simulink model "pt8612pllsimple"  (Simulink 5.0)
settings: Solver=ode45  StartTime=0.0  StopTime=10  RelTol=1e-7  AbsTol=1e-10
values from neighbouring files (symbols this model uses):
  C = 680e-9    (= 6.8e-07)    [PT8612PLLinit.m]    (also in PT8612PLLinit_2.m; PT8612PLLinit_3.m; PT8612PLLinit_4.m; colorimetry_rom.m = [[CrCgCb(1) 0 0];[0 CrCgCb(2) 0];[0 0 CrCgCb(3)]])
  fvcxo = 148.5e6/1.001    (= 148351648.352)    [PT8612PLLinit.m]    (also in PT8612PLLinit_2.m; PT8612PLLinit_3.m; PT8612PLLinit_4.m)
  Gi = 1/32    (= 0.03125)    [PT8612PLLinit.m]    (also in PT8612PLLinit_2.m = 0.05)
  Gp = 1/4    (= 0.25)    [PT8612PLLinit.m]    (also in PT8612PLLinit_2.m = 0.025; PT8612PLLinit_4.m = 256)
  Kvcxo = 90e-6    (= 9e-05)    [PT8612PLLinit.m]    (also in PT8612PLLinit_2.m; PT8612PLLinit_3.m; PT8612PLLinit_4.m)
  R = 100e3    (= 100000)    [PT8612PLLinit.m]    (also in PT8612PLLinit_2.m = 220000; PT8612PLLinit_3.m = 82000; PT8612PLLinit_4.m = 200000; combi_signal.m = [R;ones(red_heigth,spl)])
libraries: simulink x1
settings Model: LastModifiedBy=thh

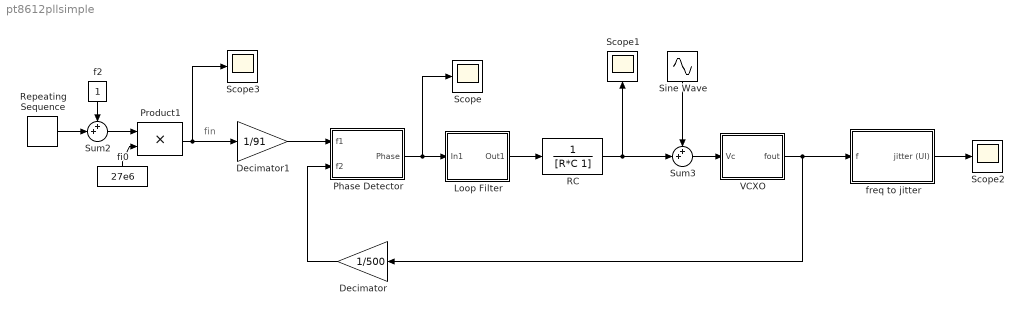
== system pt8612pllsimple ==
  note: fin
  Decimator : Gain  Orientation=left  Gain=1/500  SaturateOnIntegerOverflow=on
  Decimator1 : Gain  Gain=1/91  SaturateOnIntegerOverflow=on
  Loop Filter : Subsystem
  Phase Detector : Subsystem
  Product1 : Product  SaturateOnIntegerOverflow=on
  RC : TransferFcn  Denominator=[R*C 1]
  Repeating Sequence : simulink/Sources/Repeating Sequence  rep_seq_t=[0 1 1 10]  rep_seq_y=[0 0 1 1]*0
  Scope{,1..3} (4 alike) : Scope
      Scope settings: YMin=5.55112e-017  YMax=1.9
      Scope1 settings: Orientation=up  TimeRange=10  YMin=-0.35  YMax=0.2
      Scope2 settings: TimeRange=10  YMin=-1  YMax=0.8  SaveName=ScopeData3
      Scope3 settings: YMin=5.55112e-017  YMax=1.9  SaveName=ScopeData4
  Sine Wave : Sin  Orientation=down  Frequency=80  SampleTime=0
  Sum2 : Sum  Inputs=++|  SaturateOnIntegerOverflow=on
  Sum3 : Sum  Inputs=++|  SaturateOnIntegerOverflow=on
  VCXO : Subsystem
  f2 : Constant  Orientation=down
  fi0 : Constant  Orientation=up  Value=27e6
  freq to jitter : Subsystem
  wires:
  Phase Detector/1(Phase) -> Scope/1, Loop Filter/1(In1)
  VCXO/1(fout) -> Decimator/1, freq to jitter/1(f)
  Product1/1 -> Decimator1/1, Scope3/1
  fi0/1 -> Product1/2
  f2/1 -> Sum2/1
  Sum2/1 -> Product1/1
  Repeating Sequence/1 -> Sum2/2
  Decimator/1 -> Phase Detector/2(f2)
  Decimator1/1 -> Phase Detector/1(f1)
  Loop Filter/1(Out1) -> RC/1
  RC/1 -> Scope1/1, Sum3/2
  freq to jitter/1(jitter (UI)) -> Scope2/1
  Sum3/1 -> VCXO/1(Vc)
  Sine Wave/1 -> Sum3/1

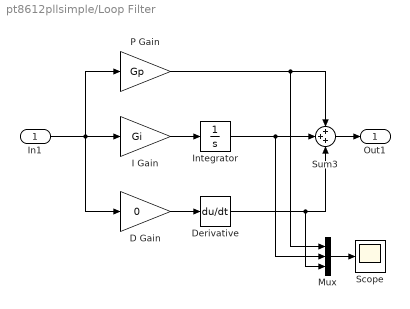
== system pt8612pllsimple/Loop Filter ==
  In1 : Inport
  D Gain : Gain  Gain=0  SaturateOnIntegerOverflow=on
  Derivative : Derivative
  I Gain : Gain  Gain=Gi  SaturateOnIntegerOverflow=on
  Integrator : Integrator
  Mux : Mux  Inputs=3
  P Gain : Gain  Gain=Gp  SaturateOnIntegerOverflow=on
  Scope : Scope
      settings: YMin=0  YMax=0.85  SaveName=ScopeData2
  Sum3 : Sum  Inputs=+++  SaturateOnIntegerOverflow=on
  Out1 : Outport
  wires:
  I Gain/1 -> Integrator/1
  P Gain/1 -> Sum3/1, Mux/1
  In1/1 -> I Gain/1, P Gain/1, D Gain/1
  Sum3/1 -> Out1/1
  D Gain/1 -> Derivative/1
  Mux/1 -> Scope/1
  Integrator/1 -> Sum3/2, Mux/2
  Derivative/1 -> Sum3/3, Mux/3

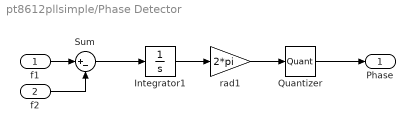
== system pt8612pllsimple/Phase Detector ==
  f1 : Inport
  f2 : Inport  Port=2
  Integrator1 : Integrator
  Quantizer : Quantizer  QuantizationInterval=2*pi/500
  Sum : Sum  Inputs=|+-  SaturateOnIntegerOverflow=on
  rad1 : Gain  Gain=2*pi  SaturateOnIntegerOverflow=on
  Phase : Outport
  wires:
  Sum/1 -> Integrator1/1
  Integrator1/1 -> rad1/1
  f1/1 -> Sum/1
  rad1/1 -> Quantizer/1
  f2/1 -> Sum/2
  Quantizer/1 -> Phase/1

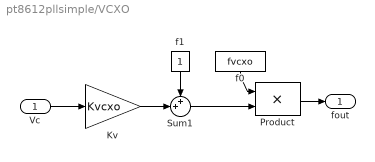
== system pt8612pllsimple/VCXO ==
  Vc : Inport
  Kv : Gain  Gain=Kvcxo  SaturateOnIntegerOverflow=on
  Product : Product  SaturateOnIntegerOverflow=on
  Sum1 : Sum  Inputs=++|  SaturateOnIntegerOverflow=on
  f0 : Constant  Orientation=down  Value=fvcxo
  f1 : Constant  Orientation=down
  fout : Outport
  wires:
  f0/1 -> Product/1
  f1/1 -> Sum1/1
  Sum1/1 -> Product/2
  Kv/1 -> Sum1/2
  Vc/1 -> Kv/1
  Product/1 -> fout/1

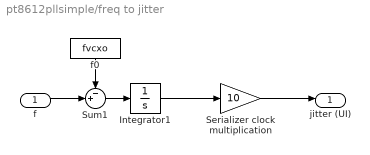
== system pt8612pllsimple/freq to jitter ==
  f : Inport
  Integrator1 : Integrator
  Serializer clock multiplication : Gain  Gain=10  SaturateOnIntegerOverflow=on
  Sum1 : Sum  Inputs=-+|  SaturateOnIntegerOverflow=on
  f0 : Constant  Orientation=down  Value=fvcxo
  jitter (UI) : Outport
  wires:
  Integrator1/1 -> Serializer clock multiplication/1
  Sum1/1 -> Integrator1/1
  f0/1 -> Sum1/1
  f/1 -> Sum1/2
  Serializer clock multiplication/1 -> jitter (UI)/1
